simulink model "HW1_2"  (R2022b)
settings: Solver=VariableStepAuto  StartTime=0.0  StopTime=9  FixedStep=0.001  MaxStep=0.001  RelTol=1e-3
values from neighbouring files (symbols this model uses):
  a_sin = [pi/2; pi/2; 0.2; pi/2]    [HW_par.m]
  Kd = 4000*eye(4)    [HW_par.m]
  Kp = 2000*eye(4)    [HW_par.m]
  omega_sin = 0.5*[1; 1; 1; 1]    [HW_par.m]
  q_0 = [0;0;0;0]    [HW_par.m]
  q_dot_0 = [0;0;0;0]    [HW_par.m]
undefined symbols (not defined in the file or in its folder): a_filt, b_filt
settings Model: Creator=Alberto  LastModifiedBy=emanuelevitetta
settings SolverCC: AlgebraicLoopSolver=TrustRegion
settings DebuggingCC: UnconnectedInputMsg=warning  UnconnectedOutputMsg=warning  UnconnectedLineMsg=warning  SFMachineParentedDataDiag=warning
settings ModelReferenceCC: EnableRefExpFcnMdlSchedulingChecks=on
settings RTWCC: DLArmComputeVersion=19.05

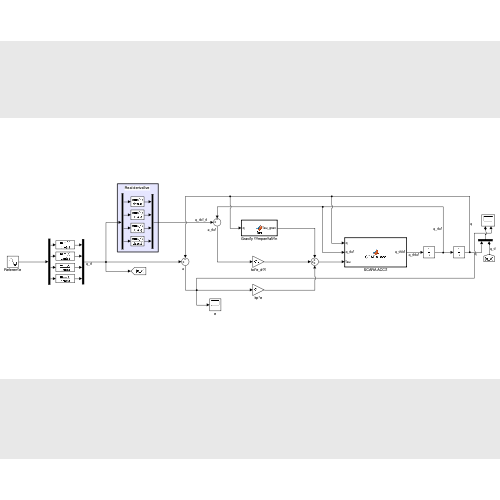
[thumbnail: Simulink's stored preview of the top-level diagram]
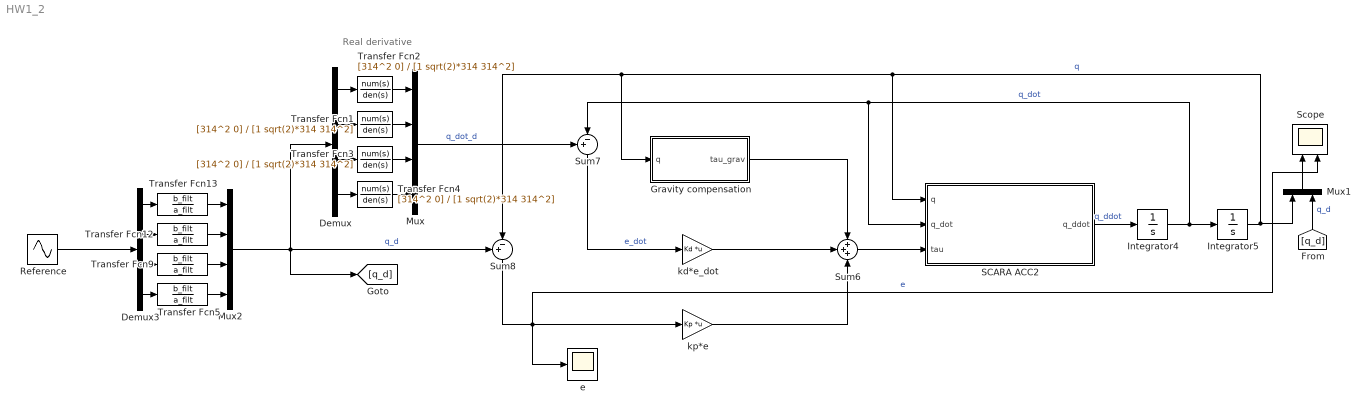
== system HW1_2 ==
  note: Real derivative
  Demux : Demux
  Demux3 : Demux
  Gravity compensation : MATLAB Function  TreatAsAtomicUnit=on
  Integrator4 : Integrator  InitialCondition=q_dot_0
  Integrator5 : Integrator  InitialCondition=q_0
  Mux : Mux
  Mux1 : Mux  Inputs=2
  Mux2 : Mux
  Reference : Sin  Amplitude=a_sin  Frequency=omega_sin  SampleTime=0.001
  SCARA ACC2 : MATLAB Function  TreatAsAtomicUnit=on
  Scope : Scope  NumInputPorts=2
  Sum6 : Sum  Inputs=+++
  Sum7 : Sum  Inputs=+-|
  Sum8 : Sum  Inputs=+-|
  Transfer Fcn{1..4} (4 alike) : TransferFcn  Numerator=[314^2 0]  Denominator=[1 sqrt(2)*314 314^2]
  Transfer Fcn{5,9,12..13} (4 alike) : TransferFcn  Numerator=b_filt  Denominator=a_filt
  e : Scope
  kd*e_dot : Gain  Gain=Kd  Multiplication=Matrix(K*u)
  kp*e : Gain  Gain=Kp  Multiplication=Matrix(K*u)
  wires:
  kd*e_dot/1 -> Sum6/2
  Mux2/1 -> [q_d], Demux/1, Sum8/1  "q_d"
  Demux3/2 -> Transfer Fcn12/1
  Transfer Fcn5/1 -> Mux2/4
  Transfer Fcn9/1 -> Mux2/3
  Demux3/1 -> Transfer Fcn13/1
  Demux3/4 -> Transfer Fcn5/1
  Mux/1 -> Sum7/1  "q_dot_d"
  Integrator5/1 -> Mux1/1, Sum8/2, Gravity compensation/1(q), SCARA ACC2/1(q)  "q"
  kp*e/1 -> Sum6/3
  Transfer Fcn2/1 -> Mux/1
  Demux3/3 -> Transfer Fcn9/1
  Sum8/1 -> e/1, Scope/2, kp*e/1  "e"
  Gravity compensation/1(tau_grav) -> Sum6/1
  Reference/1 -> Demux3/1
  Integrator4/1 -> Sum7/2, SCARA ACC2/2(q_dot), Integrator5/1  "q_dot"
  Transfer Fcn12/1 -> Mux2/2
  Sum7/1 -> kd*e_dot/1  "e_dot"
  SCARA ACC2/1(q_ddot) -> Integrator4/1  "q_ddot"
  Sum6/1 -> SCARA ACC2/3(tau)
  Transfer Fcn13/1 -> Mux2/1
  Demux/1 -> Transfer Fcn2/1
  Demux/2 -> Transfer Fcn1/1
  Transfer Fcn1/1 -> Mux/2
  Transfer Fcn3/1 -> Mux/3
  Demux/3 -> Transfer Fcn3/1
  Demux/4 -> Transfer Fcn4/1
  Transfer Fcn4/1 -> Mux/4
  [q_d] -> Mux1/2  "q_d"
  Mux1/1 -> Scope/1

== matlab function HW1_2/SCARA ACC2 ==
  data: q input; q_ddot output; q_dot input; tau input
function q_ddot = SCARA_acc(q, q_dot, tau)%#codegen
coder.extrinsic('f_B_mex'); 
coder.extrinsic('f_C_vect_mex'); 
coder.extrinsic('f_g_vect_mex');
B = eye(4);
C_vect = zeros(4,1);
F_g = zeros(4,1);
tau = reshape(tau,4,1);
q_ddot = zeros(4,1);
B = full(f_B_mex('f_B',q));
C_vect = full(f_C_vect_mex('f_C_vect', q, q_dot));
F_g = full(f_g_vect_mex('f_g_vect', q));
q_ddot = (eye(4)/B)*(-C_vect-F_g+tau);

== matlab function HW1_2/Gravity compensation ==
  data: q input; tau_grav output
function tau_grav = fcn(q)%#codegen
coder.extrinsic('f_g_vect_mex');
tau_grav = zeros(4,1);
tau_grav = reshape(full(f_g_vect_mex('f_g_vect', q)),4,1);
